simulink model "simulinkShaperTem"  (R2021b)
settings: Solver=ode3  StartTime=0.0  StopTime=1  FixedStep=0.00001  RelTol=1e-3
values from neighbouring files (symbols this model uses):
  A1 = 1 / (1 + K)    [parameter_Initial.m]
  A2 = K / (1 + K)    [parameter_Initial.m]
  td = pi / (wn * sqrt(1 - zeta^2))    [parameter_Initial.m]
  wn = 2.6968e+03    (= 2696.8)    [parameter_Initial.m]
  zeta = 0.24    [parameter_Initial.m]
settings Model: Creator=kk  LastModifiedBy=28626
settings SolverCC: AlgebraicLoopSolver=TrustRegion
settings DataIOCC: ReturnWorkspaceOutputs=off
settings DebuggingCC: SFMachineParentedDataDiag=warning  ArithmeticOperatorsInVariantConditions=warning
settings SFSimCC: SimUseLocalCustomCode=off  CustomCodeUndefinedFunction=UseInterfaceOnly
settings RTWCC: RTWUseLocalCustomCode=off

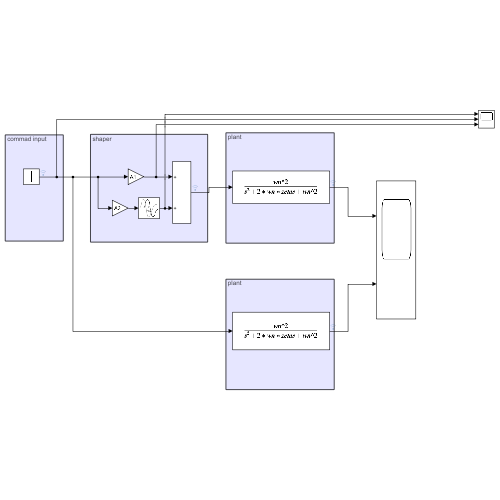
[thumbnail: Simulink's stored preview of the top-level diagram]
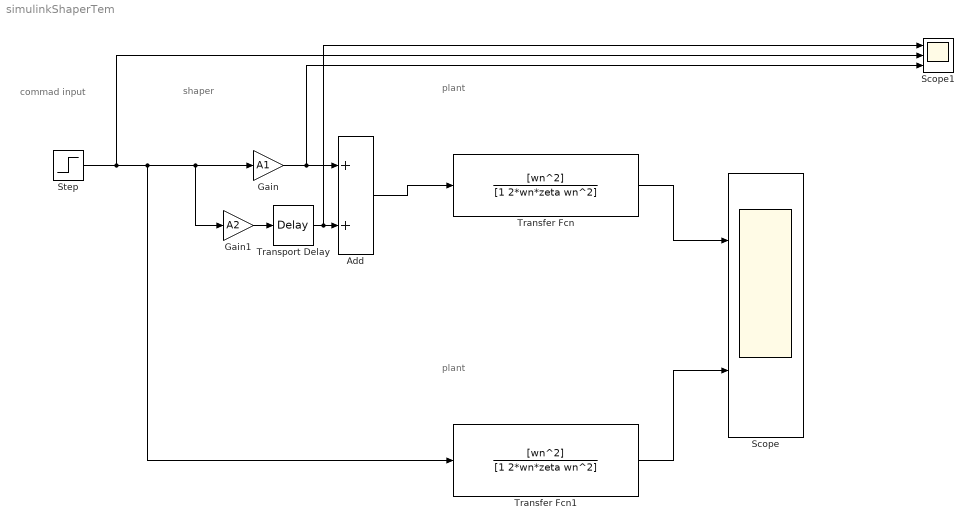
== system simulinkShaperTem ==
  note: plant
  note: commad input
  note: shaper
  note: plant
  Add : Sum
  Gain : Gain  Gain=A1
  Gain1 : Gain  Gain=A2
  Scope : Scope  NumInputPorts=2
  Scope1 : Scope  NumInputPorts=3
  Step : Step  Time=0.5  After=6  SampleTime=0
  Transfer Fcn : TransferFcn  Numerator=[wn^2]  Denominator=[1 2*wn*zeta wn^2]
  Transfer Fcn1 : TransferFcn  Numerator=[wn^2]  Denominator=[1 2*wn*zeta wn^2]
  Transport Delay : TransportDelay  DelayTime=td  PadeOrder=1
  wires:
  Transfer Fcn/1 -> Scope/1
  Transport Delay/1 -> Scope1/1, Add/2
  Gain1/1 -> Transport Delay/1
  Step/1 -> Scope1/2, Transfer Fcn1/1, Gain1/1, Gain/1
  Gain/1 -> Scope1/3, Add/1
  Add/1 -> Transfer Fcn/1
  Transfer Fcn1/1 -> Scope/2
